simulink model "stateflow2"  (R2023a)
settings: Solver=VariableStepAuto  StartTime=0.0  StopTime=10.0  RelTol=1e-3
settings Model: Creator=Administrator  LastModifiedBy=Administrator

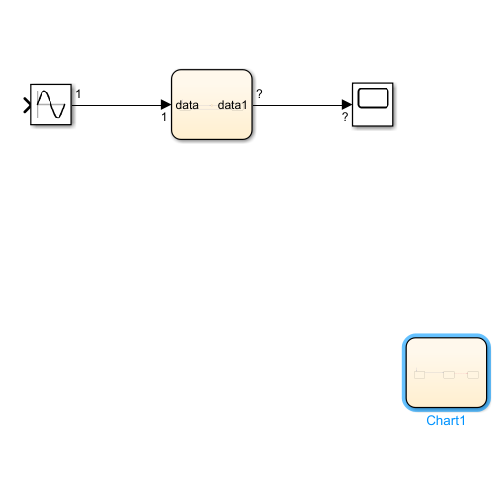
[thumbnail: Simulink's stored preview of the top-level diagram]
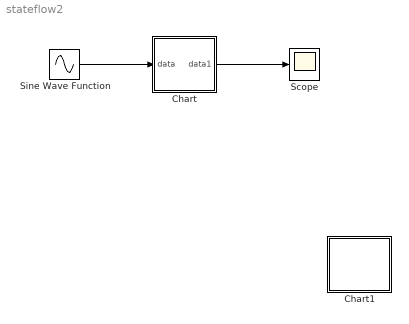
== system stateflow2 ==
  Chart : Stateflow chart  TreatAsAtomicUnit=on
  Chart1 : Stateflow chart  TreatAsAtomicUnit=on
  Scope : Scope
  Sine Wave Function : Sin  TimeSource=Use external signal  SampleTime=0
  wires:
  Sine Wave Function/1 -> Chart/1(data)
  Chart/1(data1) -> Scope/1

== stateflow chart stateflow2/Chart1 ==
  state A
    en: out = 1;
  state B
    en:out = 2;
  state ?
  (default) -> A
  A -> B : [inp  > 5]
  B -> ? : [inp > 10]

== stateflow chart stateflow2/Chart ==
  state A
    entry:
    i = 0;
    y = 0;
  state B
    entry:
    printf("this is B\r")
  (default) -> A
  A -> (junction 12) : [u > 0]{i = i + 1;}/{y=1;}
  (junction 12) -> B : [i > 10]
  B -> A
  data: data input; data1 output
